simulink model "simulacaoPioneerP3DX"  (R2023a)
settings: Solver=VariableStepAuto  StartTime=0.0  StopTime=20  RelTol=1e-3
values from neighbouring files (symbols this model uses):
  d = 44.51e-3    (= 0.04451)    [Atv01.m]
  I = Ic + mc*d^2 + 2*mw*L^2 + 2*Im    (= 0.2786255713)    [Atv01.m]
  Ic = 130.7e-3    (= 0.1307)    [Atv01.m]
  Iw = 40e-3    (= 0.04)    [Atv01.m]
  Kb = 23e-3    (= 0.023)    [Atv01.m]
  Kt = 29e-3    (= 0.029)    [Atv01.m]
  L = 0.1655    [Atv01.m]
  La = 0.66e-3    (= 0.00066)    [Atv01.m]
  m = mc + 2*mw    (= 16)    [Atv01.m]
  mc = 13    [Atv01.m]
  N = 38.3    [Atv01.m]
  R = D/2    (= 0.0975)    [Atv01.m]
  Ra = 710e-3    (= 0.71)    [Atv01.m]
settings Model: Creator=Matheus  LastModifiedBy=Matheus

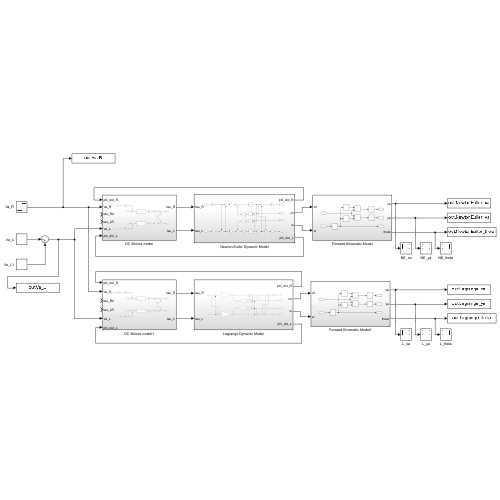
[thumbnail: Simulink's stored preview of the top-level diagram]
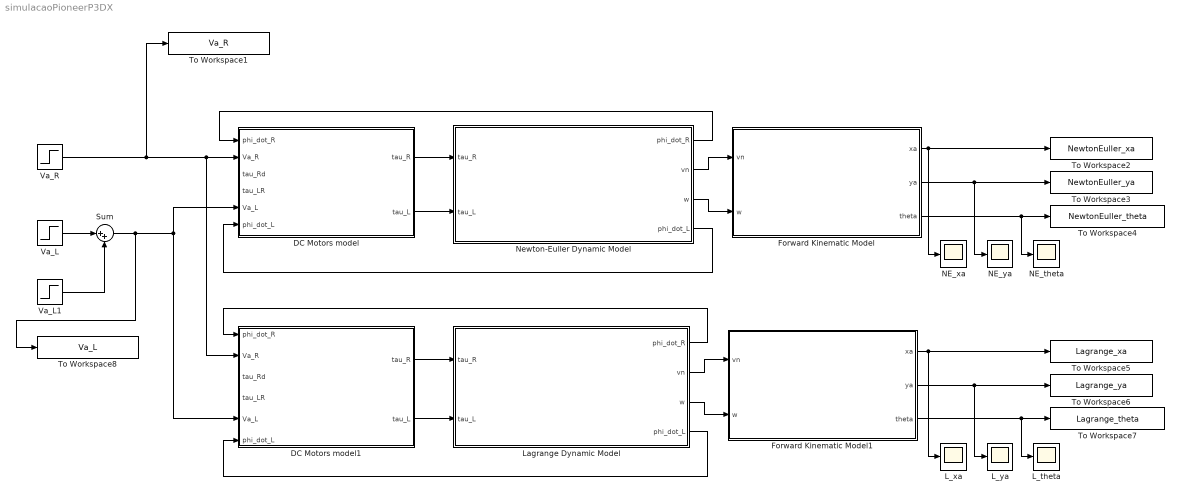
== system simulacaoPioneerP3DX ==
  DC Motors model : Subsystem
  DC Motors model1 : Subsystem
  Forward Kinematic Model : Subsystem
  Forward Kinematic Model1 : Subsystem
  L_theta : Scope
  L_xa : Scope
  L_ya : Scope
  Lagrange Dynamic Model : Subsystem
  NE_theta : Scope
  NE_xa : Scope
  NE_ya : Scope
  Newton-Euller Dynamic Model : Subsystem
  Sum : Sum  Inputs=|++
  To Workspace1 : ToWorkspace  VariableName=Va_R  SaveFormat=Structure With Time  SampleTime=-1
  To Workspace2 : ToWorkspace  VariableName=NewtonEuller_xa  SaveFormat=Structure With Time  SampleTime=-1
  To Workspace3 : ToWorkspace  VariableName=NewtonEuller_ya  SaveFormat=Structure With Time  SampleTime=-1
  To Workspace4 : ToWorkspace  VariableName=NewtonEuller_theta  SaveFormat=Structure With Time  SampleTime=-1
  To Workspace5 : ToWorkspace  VariableName=Lagrange_xa  SaveFormat=Structure With Time  SampleTime=-1
  To Workspace6 : ToWorkspace  VariableName=Lagrange_ya  SaveFormat=Structure With Time  SampleTime=-1
  To Workspace7 : ToWorkspace  VariableName=Lagrange_theta  SaveFormat=Structure With Time  SampleTime=-1
  To Workspace8 : ToWorkspace  VariableName=Va_L  SaveFormat=Structure With Time  SampleTime=-1
  Va_L : Step  Time=9.47  Before=2  After=0  SampleTime=0
  Va_L1 : Step  Time=2*9.47  After=2  SampleTime=0
  Va_R : Step  Time=9.47  After=2  SampleTime=0
  wires:
  Newton-Euller Dynamic Model/1(phi_dot_R) -> DC Motors model/1(phi_dot_R)
  Newton-Euller Dynamic Model/4(phi_dot_L) -> DC Motors model/6(phi_dot_L)
  DC Motors model/1(tau_R) -> Newton-Euller Dynamic Model/1(tau_R)
  DC Motors model/2(tau_L) -> Newton-Euller Dynamic Model/2(tau_L)
  Newton-Euller Dynamic Model/2(vn) -> Forward Kinematic Model/1(vn)
  Forward Kinematic Model/1(xa) -> NE_xa/1, To Workspace2/1
  Forward Kinematic Model/2(ya) -> NE_ya/1, To Workspace3/1
  Forward Kinematic Model/3(theta) -> NE_theta/1, To Workspace4/1
  DC Motors model1/2(tau_L) -> Lagrange Dynamic Model/2(tau_L)
  Lagrange Dynamic Model/4(phi_dot_L) -> DC Motors model1/6(phi_dot_L)
  DC Motors model1/1(tau_R) -> Lagrange Dynamic Model/1(tau_R)
  Lagrange Dynamic Model/1(phi_dot_R) -> DC Motors model1/1(phi_dot_R)
  Sum/1 -> To Workspace8/1, DC Motors model/5(Va_L), DC Motors model1/5(Va_L)
  Forward Kinematic Model1/2(ya) -> L_ya/1, To Workspace6/1
  Forward Kinematic Model1/3(theta) -> L_theta/1, To Workspace7/1
  Lagrange Dynamic Model/3(w) -> Forward Kinematic Model1/2(w)
  Forward Kinematic Model1/1(xa) -> L_xa/1, To Workspace5/1
  Lagrange Dynamic Model/2(vn) -> Forward Kinematic Model1/1(vn)
  Va_R/1 -> To Workspace1/1, DC Motors model1/2(Va_R), DC Motors model/2(Va_R)
  Newton-Euller Dynamic Model/3(w) -> Forward Kinematic Model/2(w)
  Va_L/1 -> Sum/1
  Va_L1/1 -> Sum/2

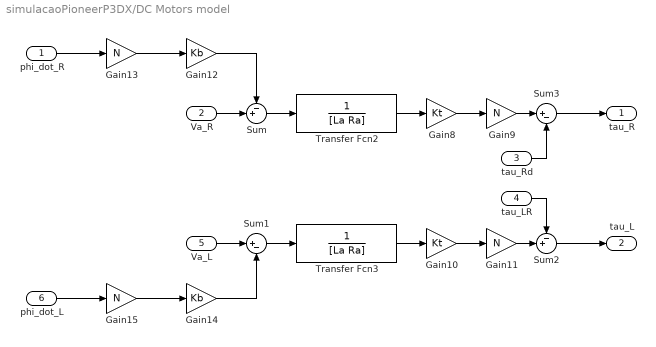
== system simulacaoPioneerP3DX/DC Motors model ==
  phi_dot_R : Inport
  Va_R : Inport  Port=2
  tau_Rd : Inport  Port=3
  tau_LR : Inport  Port=4
  Va_L : Inport  Port=5
  phi_dot_L : Inport  Port=6
  Gain10 : Gain  Gain=Kt
  Gain{9,11,13,15} (4 alike) : Gain  Gain=N
  Gain12 : Gain  Gain=Kb
  Gain14 : Gain  Gain=Kb
  Gain8 : Gain  Gain=Kt
  Sum : Sum  Inputs=-+|
  Sum1 : Sum  Inputs=|+-
  Sum2 : Sum  Inputs=-+|
  Sum3 : Sum  Inputs=|+-
  Transfer Fcn2 : TransferFcn  Denominator=[La Ra]
  Transfer Fcn3 : TransferFcn  Denominator=[La Ra]
  tau_R : Outport
  tau_L : Outport  Port=2
  wires:
  Gain8/1 -> Gain9/1
  Gain14/1 -> Sum1/2
  Gain9/1 -> Sum3/1
  Sum/1 -> Transfer Fcn2/1
  tau_LR/1 -> Sum2/1
  Gain15/1 -> Gain14/1
  Transfer Fcn2/1 -> Gain8/1
  Gain11/1 -> Sum2/2
  Gain10/1 -> Gain11/1
  Gain13/1 -> Gain12/1
  Sum1/1 -> Transfer Fcn3/1
  Gain12/1 -> Sum/1
  Transfer Fcn3/1 -> Gain10/1
  Sum3/1 -> tau_R/1
  Sum2/1 -> tau_L/1
  Va_R/1 -> Sum/2
  Va_L/1 -> Sum1/1
  tau_Rd/1 -> Sum3/2
  phi_dot_R/1 -> Gain13/1
  phi_dot_L/1 -> Gain15/1

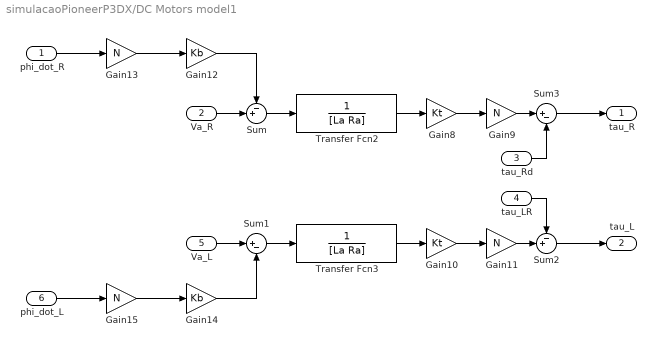
== system simulacaoPioneerP3DX/DC Motors model1 ==
  phi_dot_R : Inport
  Va_R : Inport  Port=2
  tau_Rd : Inport  Port=3
  tau_LR : Inport  Port=4
  Va_L : Inport  Port=5
  phi_dot_L : Inport  Port=6
  Gain10 : Gain  Gain=Kt
  Gain{9,11,13,15} (4 alike) : Gain  Gain=N
  Gain12 : Gain  Gain=Kb
  Gain14 : Gain  Gain=Kb
  Gain8 : Gain  Gain=Kt
  Sum : Sum  Inputs=-+|
  Sum1 : Sum  Inputs=|+-
  Sum2 : Sum  Inputs=-+|
  Sum3 : Sum  Inputs=|+-
  Transfer Fcn2 : TransferFcn  Denominator=[La Ra]
  Transfer Fcn3 : TransferFcn  Denominator=[La Ra]
  tau_R : Outport
  tau_L : Outport  Port=2
  wires:
  Gain8/1 -> Gain9/1
  Gain14/1 -> Sum1/2
  Gain9/1 -> Sum3/1
  Sum/1 -> Transfer Fcn2/1
  tau_LR/1 -> Sum2/1
  Gain15/1 -> Gain14/1
  Transfer Fcn2/1 -> Gain8/1
  Gain11/1 -> Sum2/2
  Gain10/1 -> Gain11/1
  Gain13/1 -> Gain12/1
  Sum1/1 -> Transfer Fcn3/1
  Gain12/1 -> Sum/1
  Transfer Fcn3/1 -> Gain10/1
  Sum3/1 -> tau_R/1
  Sum2/1 -> tau_L/1
  Va_R/1 -> Sum/2
  Va_L/1 -> Sum1/1
  tau_Rd/1 -> Sum3/2
  phi_dot_R/1 -> Gain13/1
  phi_dot_L/1 -> Gain15/1

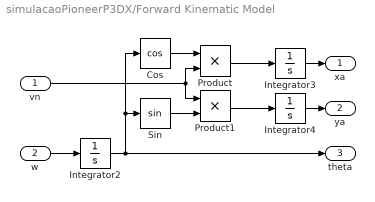
== system simulacaoPioneerP3DX/Forward Kinematic Model ==
  vn : Inport
  w : Inport  Port=2
  Cos : Trigonometry  Operator=cos
  Integrator2 : Integrator
  Integrator3 : Integrator
  Integrator4 : Integrator
  Product : Product
  Product1 : Product
  Sin : Trigonometry
  xa : Outport
  ya : Outport  Port=2
  theta : Outport  Port=3
  wires:
  Product1/1 -> Integrator4/1
  Sin/1 -> Product1/2
  Integrator3/1 -> xa/1
  Integrator4/1 -> ya/1
  Integrator2/1 -> theta/1, Cos/1, Sin/1
  Cos/1 -> Product/1
  Product/1 -> Integrator3/1
  vn/1 -> Product1/1, Product/2
  w/1 -> Integrator2/1

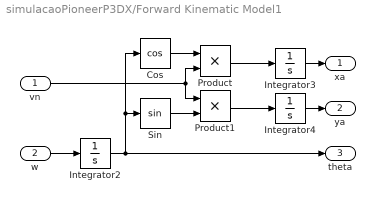
== system simulacaoPioneerP3DX/Forward Kinematic Model1 ==
  vn : Inport
  w : Inport  Port=2
  Cos : Trigonometry  Operator=cos
  Integrator2 : Integrator
  Integrator3 : Integrator
  Integrator4 : Integrator
  Product : Product
  Product1 : Product
  Sin : Trigonometry
  xa : Outport
  ya : Outport  Port=2
  theta : Outport  Port=3
  wires:
  Product1/1 -> Integrator4/1
  Sin/1 -> Product1/2
  Integrator3/1 -> xa/1
  Integrator4/1 -> ya/1
  Integrator2/1 -> theta/1, Cos/1, Sin/1
  Cos/1 -> Product/1
  Product/1 -> Integrator3/1
  vn/1 -> Product1/1, Product/2
  w/1 -> Integrator2/1

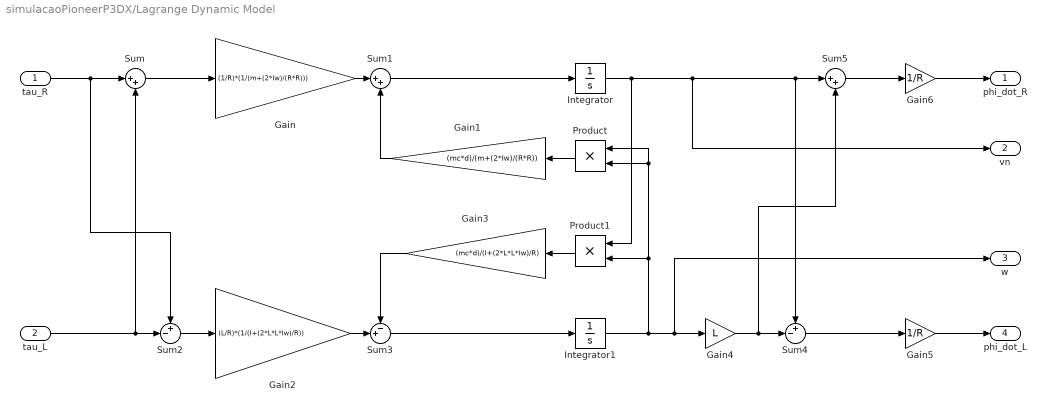
== system simulacaoPioneerP3DX/Lagrange Dynamic Model ==
  tau_R : Inport
  tau_L : Inport  Port=2
  Gain : Gain  Gain=(1/R)*(1/(m+(2*Iw)/(R*R)))
  Gain1 : Gain  Gain=(mc*d)/(m+(2*Iw)/(R*R))
  Gain2 : Gain  Gain=(L/R)*(1/(I+(2*L*L*Iw)/R))
  Gain3 : Gain  Gain=(mc*d)/(I+(2*L*L*Iw)/R)
  Gain4 : Gain  Gain=L
  Gain5 : Gain  Gain=1/R
  Gain6 : Gain  Gain=1/R
  Integrator : Integrator
  Integrator1 : Integrator
  Product : Product
  Product1 : Product
  Sum : Sum  Inputs=|++
  Sum1 : Sum  Inputs=|++
  Sum2 : Sum  Inputs=+-|
  Sum3 : Sum  Inputs=-+|
  Sum4 : Sum  Inputs=+-|
  Sum5 : Sum  Inputs=|++
  phi_dot_R : Outport
  vn : Outport  Port=2
  w : Outport  Port=3
  phi_dot_L : Outport  Port=4
  wires:
  Sum/1 -> Gain/1
  Gain4/1 -> Sum5/2, Sum4/2
  Integrator/1 -> vn/1, Sum5/1, Sum4/1, Product1/1
  Integrator1/1 -> w/1, Gain4/1, Product1/2, Product/1, Product/2
  Gain2/1 -> Sum3/2
  tau_R/1 -> Sum2/1, Sum/1
  Sum5/1 -> Gain6/1
  Product1/1 -> Gain3/1
  Sum3/1 -> Integrator1/1
  tau_L/1 -> Sum2/2, Sum/2
  Gain3/1 -> Sum3/1
  Product/1 -> Gain1/1
  Gain/1 -> Sum1/1
  Gain1/1 -> Sum1/2
  Sum4/1 -> Gain5/1
  Sum2/1 -> Gain2/1
  Sum1/1 -> Integrator/1
  Gain5/1 -> phi_dot_L/1
  Gain6/1 -> phi_dot_R/1

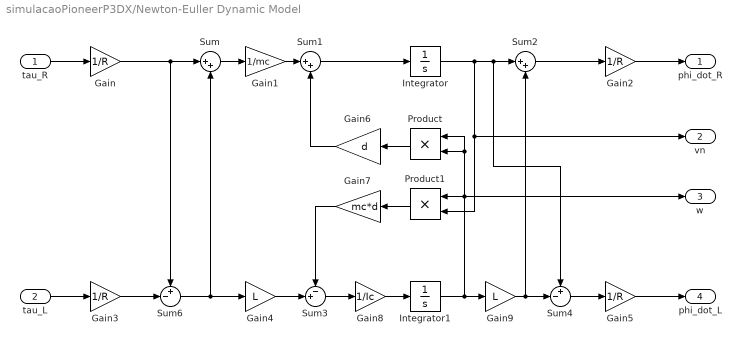
== system simulacaoPioneerP3DX/Newton-Euller Dynamic Model ==
  tau_R : Inport
  tau_L : Inport  Port=2
  Gain{,2..3,5} (4 alike) : Gain  Gain=1/R
  Gain1 : Gain  Gain=1/mc
  Gain4 : Gain  Gain=L
  Gain6 : Gain  Gain=d
  Gain7 : Gain  Gain=mc*d
  Gain8 : Gain  Gain=1/Ic
  Gain9 : Gain  Gain=L
  Integrator : Integrator
  Integrator1 : Integrator
  Product : Product
  Product1 : Product
  Sum : Sum  Inputs=|++
  Sum1 : Sum  Inputs=|++
  Sum2 : Sum  Inputs=|++
  Sum3 : Sum  Inputs=-+|
  Sum4 : Sum  Inputs=+-|
  Sum6 : Sum  Inputs=+-|
  phi_dot_R : Outport
  vn : Outport  Port=2
  w : Outport  Port=3
  phi_dot_L : Outport  Port=4
  wires:
  Sum4/1 -> Gain5/1
  Integrator/1 -> vn/1, Product1/2, Sum4/1, Sum2/1
  Integrator1/1 -> Gain9/1, w/1, Product/2, Product/1, Product1/1
  Sum6/1 -> Gain4/1, Sum/2
  Gain4/1 -> Sum3/2
  Sum/1 -> Gain1/1
  Gain3/1 -> Sum6/2
  Gain1/1 -> Sum1/1
  Sum2/1 -> Gain2/1
  Gain9/1 -> Sum4/2, Sum2/2
  Product1/1 -> Gain7/1
  Gain/1 -> Sum/1, Sum6/1
  tau_L/1 -> Gain3/1
  Sum1/1 -> Integrator/1
  Sum3/1 -> Gain8/1
  Gain8/1 -> Integrator1/1
  Product/1 -> Gain6/1
  Gain6/1 -> Sum1/2
  Gain2/1 -> phi_dot_R/1
  tau_R/1 -> Gain/1
  Gain5/1 -> phi_dot_L/1
  Gain7/1 -> Sum3/1
